simulink model "Five_PMSM_control"  (R2014b)
settings: Solver=ode23tb  SolverMode=SingleTasking  StartTime=0.0  StopTime=0.1  FixedStep=Ts  RelTol=1e-4
undefined symbols (not defined in the file or in its folder): Ts
libraries: powerlib x6
Description:
  | Copyright 2008-2014 The MathWorks, Inc.
settings Model: ExtModeTrigMode=oneshot  ExtModeArmWhenConnect=off  ExtModeAutoUpdateStatusClock=off  Creator=MathWorks  LastModifiedBy=Lei
settings DataIOCC: ExternalInput=[]  LimitDataPoints=off  SignalLoggingSaveFormat=ModelDataLogs  SaveOutput=off  SignalLogging=off  SaveTime=off  SignalLoggingName=sigsOut
settings OptimizationCC: BlockReduction=off  BooleanDataType=off  ExpressionDepthLimit=2147483647  InitFltsAndDblsToZero=on  EfficientMapNaN2IntZero=off
settings DebuggingCC: UnderspecifiedInitializationDetection=Classic  MergeDetectMultiDrivingBlocksExec=none  CheckExecutionContextPreStartOutputMsg=on  CheckExecutionContextRuntimeOutputMsg=on  SignalResolutionControl=TryResolveAllWithWarning  SolverPrmCheckMsg=none  MultiTaskDSMMsg=warning  MultiTaskCondExecSysMsg=none  SigSpecEnsureSampleTimeMsg=none  FcnCallInpInsideContextMsg=UseLocalSettings  StateNameClashWarn=warning
settings HardwareCC: TargetUnknown=on
settings RTWCC: IncludeERTFirstTime=on
settings GRTTargetCC: CombineOutputUpdateFcns=off  GRTInterface=on

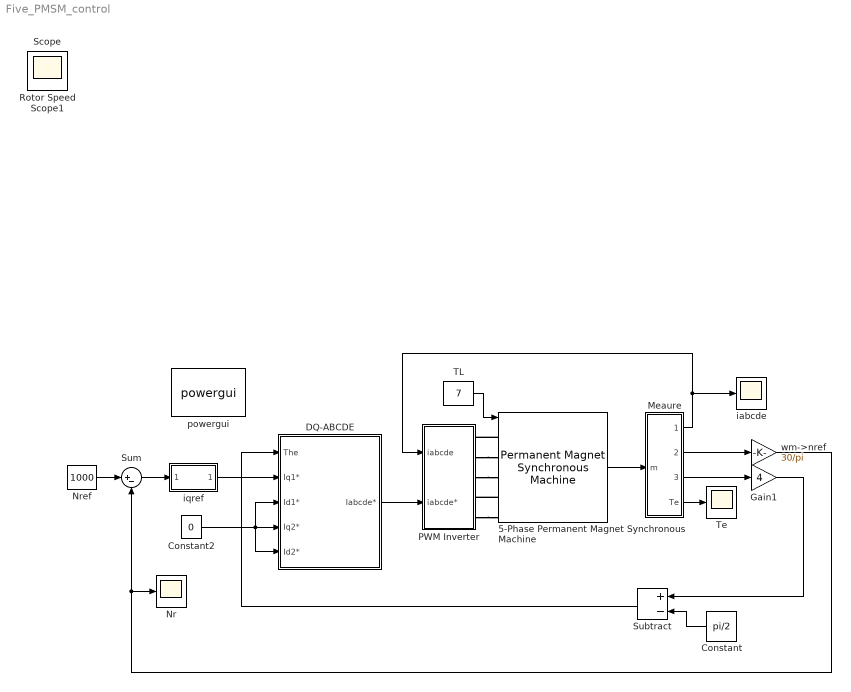
== system Five_PMSM_control ==
  5-Phase Permanent Magnet Synchronous Machine : powerlib/Machines/Permanent Magnet Synchronous Machine  NbPhases=5  FluxDistribution=Sinusoidal  RotorType=Round  MechanicalLoad=Torque Tm  PresetModel=No  ShowDetailedParameters=on  MeasurementBus=on  Resistance=0.12  Inductance=8.5e-3  dqInductances=[8.5e-3,8.5e-3]  La=1350e-6  MachineConstant=Flux linkage established by magnets (V.s)  Flux=0.05  VoltageCst=24.6211  TorqueCst=0.5  Flat=120  Mechanical=[0.002 0.02 4]  PolePairs=4  InitialConditions=[0,0, 0,0]  InitialConditions5ph=[0 0 0 0 0 0]  TsPowergui=0  TsBlock=-1  RefAngle=90 degrees behind phase A axis (modified Park)
  Constant : Constant  Value=pi/2
  Constant2 : Constant  Value=0
  DQ-ABCDE : Subsystem
  Gain1 : Gain  Gain=4  SaturateOnIntegerOverflow=on  OutDataTypeStr=Inherit: Same as input  ParamDataTypeStr=Inherit: Same as input
  Meaure : Subsystem
  Nr : Scope
      settings: YMin=200  YMax=1200  SaveName=Nr  ScrollMode=on
  Nref : Constant  Value=1000
  PWM Inverter : Subsystem
  Subtract : Sum  Inputs=+-
  Sum : Sum  Inputs=|+-
  TL : Constant  Value=7
  Te : Scope
      settings: YMin=-200  YMax=200  SaveName=Te  ScrollMode=on
  iabcde : Scope
      settings: YMin=-200  YMax=200  SaveName=iabcde  ScrollMode=on
  iqref : Subsystem  mask(PI Controller){I=1, P=3, sat=[-150, 150]}
      mask prompts: I "Integral"; P "Proportional:"; sat "Minimum and maximum outputs:"
      mask init:
      | min=sat(1);max=sat(2);
      mask Display: disp('PI')
  powergui : powerlib/powergui  SimulationMode=Continuous  SolverType=Tustin  SampleTime=Ts  frequency=60  SPID=on  DisableSnubberDevices=off  DisableRonSwitches=off  DisableVfSwitches=off  SwTol=0  DisplayEquations=off  Interpol=off  methode=off  Ts=0  frequencyindice=0  Pbase=100e6  ErrMax=1e-4  Iterations=50  UnitsV=kV  UnitsW=MW  FunctionMessages=off  echomessages=off  HookPort=off  EnableUseOfTLC=off  x0status=blocks  RestoreLinks=warning  ResistiveCurrentMeasurement=off  Frange=[0:2:500]  Ylog=off  Xlog=on  ShowGrid=off  save=off  variable=ZData  structure=0  ZoomFFT=on  StartTime=0.0  cycles=1  DisplayStyle=1  fundamental=60  FreqAxis=off  MaxFrequency=1000  frequencyindicesteady=1  RmsSteady=1  display=off
  wm->nref : Gain  Gain=30/pi  SaturateOnIntegerOverflow=on  OutDataTypeStr=Inherit: Same as input  ParamDataTypeStr=Inherit: Same as input
  Rotor Speed : Scope  NumInputPorts=2
      settings: YMin=-5~-5  YMax=5~5  ScrollMode=on
  Scope : Scope  NumInputPorts=2
      settings: YMin=-5~-5  YMax=5~5  ScrollMode=on
  Scope1 : Scope  NumInputPorts=2
      settings: YMin=-5~-5  YMax=5~5  SaveName=ScopeData2  ScrollMode=on
  wires:
  Sum/1 -> iqref/1(In_1)
  Nref/1 -> Sum/1
  wm->nref/1 -> Nr/1, Sum/2
  iqref/1(Out_1) -> DQ-ABCDE/2("Iq1* ")
  Constant2/1 -> DQ-ABCDE/3("Id1* "), DQ-ABCDE/5(Id2*), DQ-ABCDE/4(Iq2*)
  DQ-ABCDE/1(Iabcde*) -> PWM Inverter/2(iabcde*)
  TL/1 -> 5-Phase Permanent Magnet Synchronous Machine/1
  Subtract/1 -> DQ-ABCDE/1(The)
  Constant/1 -> Subtract/2
  Gain1/1 -> Subtract/1
  Meaure/1(Iabcde) -> iabcde/1, PWM Inverter/1(iabcde)
  5-Phase Permanent Magnet Synchronous Machine/1 -> Meaure/1(m)
  Meaure/2(wm) -> wm->nref/1
  Meaure/3(The) -> Gain1/1
  Meaure/4(Te) -> Te/1
  connections:
  PWM Inverter/RConn2 -- 5-Phase Permanent Magnet Synchronous Machine/LConn2
  PWM Inverter/RConn3 -- 5-Phase Permanent Magnet Synchronous Machine/LConn3
  5-Phase Permanent Magnet Synchronous Machine/LConn1 -- PWM Inverter/RConn1
  5-Phase Permanent Magnet Synchronous Machine/LConn4 -- PWM Inverter/RConn4
  PWM Inverter/RConn5 -- 5-Phase Permanent Magnet Synchronous Machine/LConn5

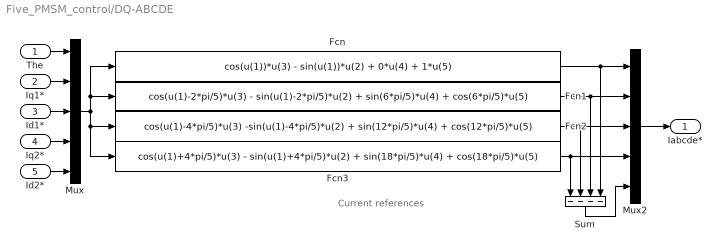
== system Five_PMSM_control/DQ-ABCDE ==
  note: Current references
  The : Inport
  "Iq1* " : Inport  Port=2
  "Id1* " : Inport  Port=3
  Iq2* : Inport  Port=4
  Id2* : Inport  Port=5
  Fcn : Fcn  Expr=cos(u(1))*u(3) - sin(u(1))*u(2) + 0*u(4) + 1*u(5)
  Fcn1 : Fcn  Expr=cos(u(1)-2*pi/5)*u(3) - sin(u(1)-2*pi/5)*u(2) + sin(6*pi/5)*u(4) + cos(6*pi/5)*u(5)
  Fcn2 : Fcn  Expr=cos(u(1)-4*pi/5)*u(3) -sin(u(1)-4*pi/5)*u(2) + sin(12*pi/5)*u(4) + cos(12*pi/5)*u(5)
  Fcn3 : Fcn  Expr=cos(u(1)+4*pi/5)*u(3) - sin(u(1)+4*pi/5)*u(2) + sin(18*pi/5)*u(4) + cos(18*pi/5)*u(5)
  Mux : Mux  Inputs=5
  Mux2 : Mux  Inputs=5
  Sum : Sum  Inputs=----  SaturateOnIntegerOverflow=on  InputSameDT=on  OutDataTypeStr=Inherit: Same as first input
  Iabcde* : Outport  InitialOutput=0
  wires:
  Sum/1 -> Mux2/5
  Fcn1/1 -> Mux2/2, Sum/3
  Fcn2/1 -> Mux2/3, Sum/2
  Fcn3/1 -> Mux2/4, Sum/1
  Mux/1 -> Fcn2/1, Fcn3/1, Fcn/1, Fcn1/1
  Fcn/1 -> Sum/4, Mux2/1
  The/1 -> Mux/1
  "Iq1* "/1 -> Mux/2
  "Id1* "/1 -> Mux/3
  Iq2*/1 -> Mux/4
  Id2*/1 -> Mux/5
  Mux2/1 -> Iabcde*/1

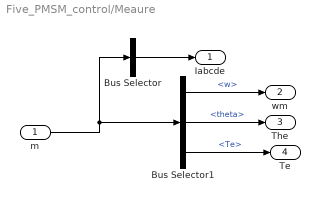
== system Five_PMSM_control/Meaure ==
  m : Inport
  Bus Selector : BusSelector  OutputSignals=ias,ibs,ics,ids,ies  OutputAsBus=on
  Bus Selector1 : BusSelector  OutputSignals=w,theta,Te
  Iabcde : Outport
  wm : Outport  Port=2
  The : Outport  Port=3
  Te : Outport  Port=4
  wires:
  Bus Selector1/1 -> wm/1  "<w>"
  Bus Selector1/2 -> The/1  "<theta>"
  m/1 -> Bus Selector/1, Bus Selector1/1
  Bus Selector1/3 -> Te/1  "<Te>"
  Bus Selector/1 -> Iabcde/1

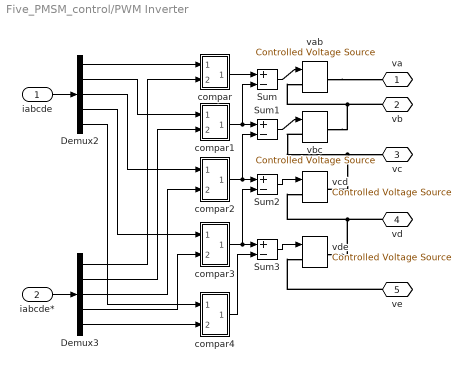
== system Five_PMSM_control/PWM Inverter ==
  iabcde : Inport
  iabcde* : Inport  Port=2
  Demux2 : Demux  Outputs=5
  Demux3 : Demux  Outputs=5
  Sum{,1..3} (4 alike) : Sum  Inputs=+-  SaturateOnIntegerOverflow=on  InputSameDT=on  OutDataTypeStr=Inherit: Same as first input
  compar : Subsystem
  compar1 : Subsystem
  compar2 : Subsystem
  compar3 : Subsystem
  compar4 : Subsystem
  vab : powerlib/Electrical Sources/Controlled Voltage Source  Description=source block  Initialize=on  Source_Type=AC  Amplitude=0  Phase=0  Frequency=0  Measurements=None
      settings: AttributesFormatString=\n
  vbc : powerlib/Electrical Sources/Controlled Voltage Source  Description=source block  Initialize=on  Source_Type=AC  Amplitude=0  Phase=0  Frequency=0  Measurements=None
      settings: AttributesFormatString=\n
  vcd : powerlib/Electrical Sources/Controlled Voltage Source  Description=source block  Initialize=on  Source_Type=AC  Amplitude=0  Phase=0  Frequency=0  Measurements=None
      settings: AttributesFormatString=\n
  vde : powerlib/Electrical Sources/Controlled Voltage Source  Description=source block  Initialize=on  Source_Type=AC  Amplitude=0  Phase=0  Frequency=0  Measurements=None
      settings: AttributesFormatString=\n
  va : PMIOPort  Port=1  Side=Right
  vb : PMIOPort  Port=2  Side=Right
  vc : PMIOPort  Port=3  Side=Right
  vd : PMIOPort  Port=4  Side=Right
  ve : PMIOPort  Port=5  Side=Right
  wires:
  Demux2/1 -> compar/1(ia)
  Demux2/2 -> compar1/1(ib)
  Demux2/3 -> compar2/1(ic)
  Demux3/3 -> compar2/2(ic*)
  Demux3/2 -> compar1/2(ib*)
  Demux3/1 -> compar/2(ia*)
  compar/1(va) -> Sum/1
  compar1/1(vb) -> Sum/2, Sum1/1
  compar2/1(vc) -> Sum1/2, Sum2/1
  iabcde/1 -> Demux2/1
  iabcde*/1 -> Demux3/1
  Sum/1 -> vab/1
  Sum1/1 -> vbc/1
  Sum2/1 -> vcd/1
  Demux3/5 -> compar4/2(ie*)
  Demux3/4 -> compar3/2(id*)
  Demux2/4 -> compar3/1(id)
  Demux2/5 -> compar4/1(ie)
  Sum3/1 -> vde/1
  compar3/1(vd) -> Sum3/1, Sum2/2
  compar4/1(ve) -> Sum3/2
  connections:
  vab/RConn1 -- va/RConn1
  vb/RConn1 -- vab/LConn1 -- vbc/RConn1
  vbc/LConn1 -- vc/RConn1 -- vcd/RConn1
  vd/RConn1 -- vcd/LConn1 -- vde/RConn1
  ve/RConn1 -- vde/LConn1

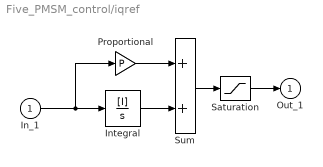
== system Five_PMSM_control/iqref ==
  In_1 : Inport
  Integral : TransferFcn  Numerator=[I]  Denominator=[1 0]
  Proportional : Gain  Gain=P  SaturateOnIntegerOverflow=on  OutDataTypeStr=Inherit: Same as input  ParamDataTypeStr=Inherit: Same as input
  Saturation : Saturate  UpperLimit=max  LowerLimit=min
  Sum : Sum  SaturateOnIntegerOverflow=on  InputSameDT=on  OutDataTypeStr=Inherit: Same as first input
  Out_1 : Outport  InitialOutput=0
  wires:
  Integral/1 -> Sum/2
  In_1/1 -> Integral/1, Proportional/1
  Proportional/1 -> Sum/1
  Sum/1 -> Saturation/1
  Saturation/1 -> Out_1/1

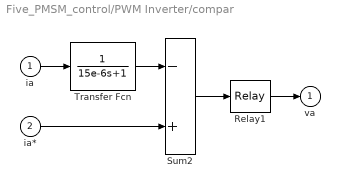
== system Five_PMSM_control/PWM Inverter/compar ==
  ia : Inport
  ia* : Inport  Port=2
  Relay1 : Relay  OnSwitchValue=0.1  OffSwitchValue=-0.1  OnOutputValue=155  OffOutputValue=-155
  Sum2 : Sum  Inputs=-+  SaturateOnIntegerOverflow=on  InputSameDT=on  OutDataTypeStr=Inherit: Same as first input
  Transfer Fcn : TransferFcn  Denominator=[15e-6 1]
  va : Outport  InitialOutput=0
  wires:
  ia*/1 -> Sum2/2
  Sum2/1 -> Relay1/1
  Relay1/1 -> va/1
  ia/1 -> Transfer Fcn/1
  Transfer Fcn/1 -> Sum2/1

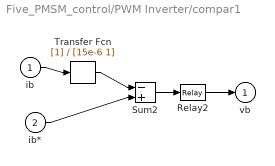
== system Five_PMSM_control/PWM Inverter/compar1 ==
  ib : Inport
  ib* : Inport  Port=2
  Relay2 : Relay  OnSwitchValue=0.1  OffSwitchValue=-0.1  OnOutputValue=155  OffOutputValue=-155
  Sum2 : Sum  Inputs=-+  SaturateOnIntegerOverflow=on  InputSameDT=on  OutDataTypeStr=Inherit: Same as first input
  Transfer Fcn : TransferFcn  Denominator=[15e-6 1]
  vb : Outport  InitialOutput=0
  wires:
  ib*/1 -> Sum2/2
  Sum2/1 -> Relay2/1
  Relay2/1 -> vb/1
  ib/1 -> Transfer Fcn/1
  Transfer Fcn/1 -> Sum2/1

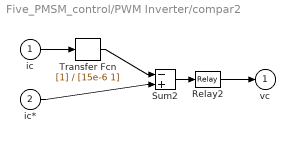
== system Five_PMSM_control/PWM Inverter/compar2 ==
  ic : Inport
  ic* : Inport  Port=2
  Relay2 : Relay  OnSwitchValue=0.1  OffSwitchValue=-0.1  OnOutputValue=155  OffOutputValue=-155
  Sum2 : Sum  Inputs=-+  SaturateOnIntegerOverflow=on  InputSameDT=on  OutDataTypeStr=Inherit: Same as first input
  Transfer Fcn : TransferFcn  Denominator=[15e-6 1]
  vc : Outport  InitialOutput=0
  wires:
  ic*/1 -> Sum2/2
  Sum2/1 -> Relay2/1
  Relay2/1 -> vc/1
  ic/1 -> Transfer Fcn/1
  Transfer Fcn/1 -> Sum2/1

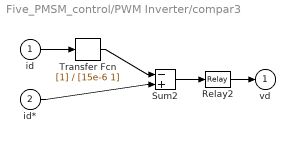
== system Five_PMSM_control/PWM Inverter/compar3 ==
  id : Inport
  id* : Inport  Port=2
  Relay2 : Relay  OnSwitchValue=0.1  OffSwitchValue=-0.1  OnOutputValue=155  OffOutputValue=-155
  Sum2 : Sum  Inputs=-+  SaturateOnIntegerOverflow=on  InputSameDT=on  OutDataTypeStr=Inherit: Same as first input
  Transfer Fcn : TransferFcn  Denominator=[15e-6 1]
  vd : Outport  InitialOutput=0
  wires:
  Transfer Fcn/1 -> Sum2/1
  id/1 -> Transfer Fcn/1
  Relay2/1 -> vd/1
  Sum2/1 -> Relay2/1
  id*/1 -> Sum2/2

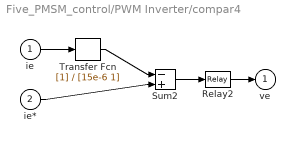
== system Five_PMSM_control/PWM Inverter/compar4 ==
  ie : Inport
  ie* : Inport  Port=2
  Relay2 : Relay  OnSwitchValue=0.1  OffSwitchValue=-0.1  OnOutputValue=155  OffOutputValue=-155
  Sum2 : Sum  Inputs=-+  SaturateOnIntegerOverflow=on  InputSameDT=on  OutDataTypeStr=Inherit: Same as first input
  Transfer Fcn : TransferFcn  Denominator=[15e-6 1]
  ve : Outport  InitialOutput=0
  wires:
  ie*/1 -> Sum2/2
  Sum2/1 -> Relay2/1
  Relay2/1 -> ve/1
  ie/1 -> Transfer Fcn/1
  Transfer Fcn/1 -> Sum2/1
